simulink model "ADC_RoadRunner"  (R2024b)
settings: Solver=ode23tb  StartTime=0  StopTime=20  FixedStep=0.01  RelTol=1e-3
model workspace (MAT data in the model file):
  finalint = 0
  firstWarning = 1
  originalScenarioChecksum = '114339432DE22364D47BB28FC96DC10C'
undefined symbols (not defined in the file): curvature, DefaultGear, Defined, DEND_B, DEND_S, DEND_T, direction, DiscIntNeverNeededParam, driving, dspblkCoreblockFVToolHelper, Ego, fractalcoef, gcbh, gradbp, L, Lane, LF, LR, m, MAX_BRAKE, MAX_STEER, MAX_TORQUE, maxNumActors, MCAR, MIN_BRAKE, MIN_STEER, MIN_TORQUE, n, NUMD_B, NUMD_S, NUMD_T, Pose, psi_o, R, RRdamp, sigbuilder_block, STEER_RATIO, Tdead, thetaRefs, TrackWidth, ts, Ts, User, Vdead, Velocity, WB, xRef2s, yRef2s
libraries: simulink x9, roadrunnerscenario x7, simulink_extras x4, drivingscenarioandsensors x3, sensorinslib x2, robotalgslib x1, mpcadaslib x1, drivingvehiclecontroller x1, slpidlib x1, sensorgpslib x1, mspsensorlib x1, LaneDetection x1
(part 1 of 4)
settings Model: Creator=akshran  LastModifiedBy=austi
settings OptimizationCC: ReuseModelBlockBuffer=off
settings DebuggingCC: UnconnectedInputMsg=warning  UnconnectedOutputMsg=warning  UnconnectedLineMsg=warning  UnderSpecifiedDimensionMsg=warning
settings ModelReferenceCC: EnableRefExpFcnMdlSchedulingChecks=on
settings RTWCC: GPUComputeCapability=3.5  DLArmComputeVersion=19.05

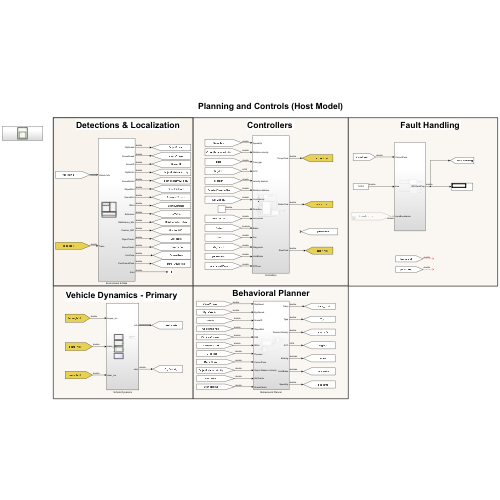
[thumbnail: Simulink's stored preview of the top-level diagram]
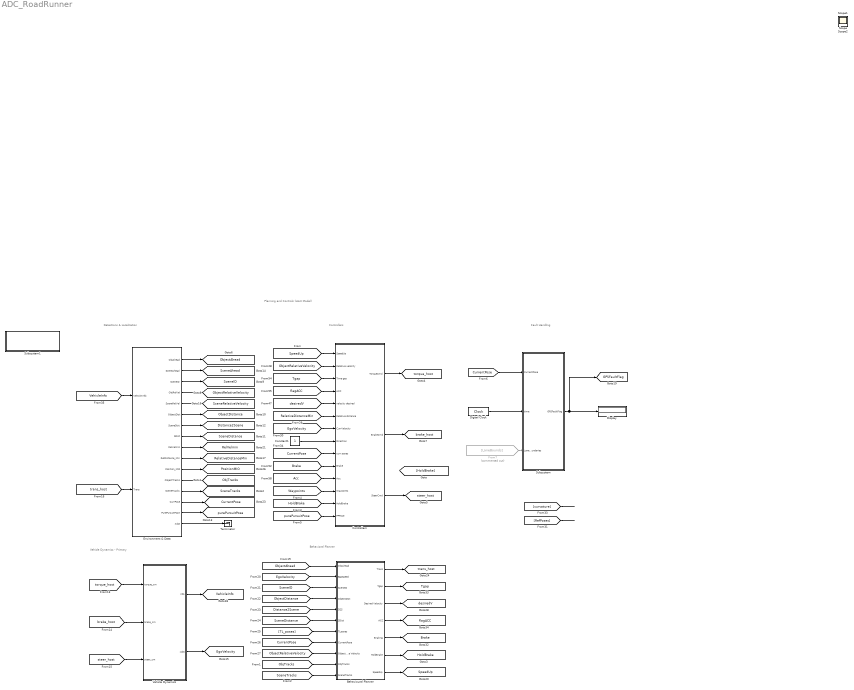
== system ADC_RoadRunner ==
  note: Planning and Controls (Host Model)
  note: Vehicle Dynamics - Primary
  note: Behavioral Planner
  note: Fault Handling
  note: Detections & Localization
  note: Controllers
  Behavioural Planner : Subsystem
  Constant1 : Constant
  Controllers : Subsystem
  Digital Clock : DigitalClock  SampleTime=Ts
  Display : Display
  Environment & Data : Subsystem
  From7 : From  Commented=on  GotoTag=LaneBounds  TagVisibility=global
  Subsystem : Subsystem
  Subsystem1 : Subsystem
  Terminator : Terminator
  Vehicle Dynamics : Subsystem
  Scope : Scope
  Scope1 : Scope
  Scope2 : Scope
  tag scope: Brake=global, CurrentPose=global, Distance2Scene=global, EgoVelocity=global, GPSFaultFlag=global, HoldBrake=global, ObjTracks=global, ObjectAhead=global, ObjectDistance=global, ObjectRelativeVelocity=global, PositionMIO=global, RelVelmin=global, RelativeDistanceMin=global, SceneAhead=global, SceneDistance=global, SceneID=global, SceneRelativeVelocity=global, SceneTracks=global, SpeedUp=global, Tgap=global, VehicleInfo=global, brake_host=global, desiredV=global, flagACC=global, purePursuitPose=global, steer_host=global, torque_host=global, trans_host=global
  wires:
  Controllers/1(TorqueCmd) -> [torque_host]
  Vehicle Dynamics/2(xdot) -> [EgoVelocity]
  Vehicle Dynamics/1(Info) -> [VehicleInfo]
  [torque_host] -> Vehicle Dynamics/1(torque_cm)
  [brake_host] -> Vehicle Dynamics/2(brake_cm)
  [steer_host] -> Vehicle Dynamics/3(steer_cm)
  [trans_host] -> Environment & Data/2(Trans)
  [ObjectRelativeVelocity] -> Controllers/2(Relative velocity)
  [RelativeDistanceMin] -> Controllers/6(Relative distance)
  [EgoVelocity] -> Controllers/7(CurrVelocity)
  [RefPoses] -> ?
  Constant1/1 -> Controllers/8(Direction)
  [curvature] -> ?
  [CurrentPose] -> Controllers/9(curr poses)
  [VehicleInfo] -> Environment & Data/1(Vehicle Info)
  [desiredV] -> Controllers/5(velocity desired)
  [Tgap] -> Controllers/3(Time gap)
  [flagACC] -> Controllers/4(ACC)
  Controllers/2(BrakeCmd) -> [brake_host]
  Controllers/3(SteerCmd) -> [steer_host]
  [ObjectAhead] -> Behavioural Planner/1(ObjAhead)
  [EgoVelocity] -> Behavioural Planner/2(EgoSpeed)
  [SceneID] -> Behavioural Planner/3(SceneID)
  [ObjectDistance] -> Behavioural Planner/4(ObjectDist)
  [Distance2Scene] -> Behavioural Planner/5(D2S)
  [SceneDistance] -> Behavioural Planner/6(SDist)
  [TL_poses] -> Behavioural Planner/7(TLposes)
  [CurrentPose] -> Behavioural Planner/8(CurrentPose)
  [ObjectRelativeVelocity] -> Behavioural Planner/9(Object Relative Velocity)
  Behavioural Planner/1(Trans) -> [trans_host]
  Behavioural Planner/2(Tgap) -> [Tgap]
  Behavioural Planner/3(Desired Velocity) -> [desiredV]
  Behavioural Planner/4(ACC) -> [flagACC]
  Behavioural Planner/5(Braking) -> [Brake]
  [Brake] -> Controllers/10(Brake)
  [Acc] -> Controllers/11(Acc)
  [ObjTracks] -> Behavioural Planner/10(ObjTracks)
  [SceneTracks] -> Behavioural Planner/11(SceneTracks)
  Behavioural Planner/6(HoldBrake) -> [HoldBrake]
  [HoldBrake] -> Controllers/13(HoldBrake)
  [Waypoints] -> Controllers/12(Waypoints)
  Behavioural Planner/7(SpeedUp) -> [SpeedUp]
  [SpeedUp] -> Controllers/1(SpeedUp)
  [purePursuitPose] -> Controllers/14(PPPose)
  [CurrentPose] -> Subsystem/1(CurrentPose)
  Digital Clock/1 -> Subsystem/2(time)
  Subsystem/1(GPSFaultFlag) -> Display/1, [GPSFaultFlag]
  Environment & Data/1(ObjAhead) -> [ObjectAhead]
  Environment & Data/4(ObjRelVel) -> [ObjectRelativeVelocity]
  Environment & Data/3(SceneID) -> [SceneID]
  Environment & Data/6(ObjectDist) -> [ObjectDistance]
  Environment & Data/7(SceneDist) -> [Distance2Scene]
  Environment & Data/8(SDist) -> [SceneDistance]
  Environment & Data/10(RelDistance_Min) -> [RelativeDistanceMin]
  Environment & Data/15(PurePursuitPose) -> [purePursuitPose]
  Environment & Data/14(CurrPose) -> [CurrentPose]
  Environment & Data/12(ObjectTracks) -> [ObjTracks]
  Environment & Data/13(SceneTracks) -> [SceneTracks]
  Environment & Data/11(Position_MIO) -> [PositionMIO]
  Environment & Data/2(SceneAhead) -> [SceneAhead]
  Environment & Data/9(RelVelmin) -> [RelVelmin]
  Environment & Data/5(SceneRelVel) -> [SceneRelativeVelocity]
  Environment & Data/16(Xdot) -> Terminator/1
  From7/1 -> Subsystem/3(LaneBoundaries)

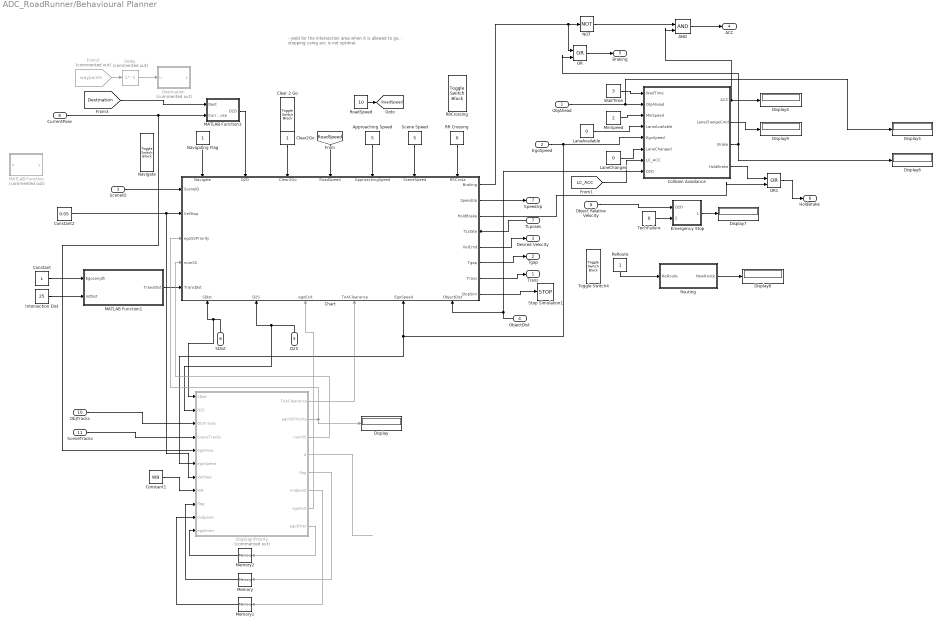
== system ADC_RoadRunner/Behavioural Planner ==
  note: - yield for the intersection area when it is allowed to go.
      | - stopping using acc is not optimal.
  ObjAhead : Inport
  EgoSpeed : Inport  Port=2
  SceneID : Inport  Port=3
  ObjectDist : Inport  Port=4
  D2S : Inport  Port=5
  SDist : Inport  Port=6
  TLposes : Inport  Port=7
  CurrentPose : Inport  Port=8
  Object Relative Velocity : Inport  Port=9
  ObjTracks : Inport  Port=10
  SceneTracks : Inport  Port=11
  AND : Logic  IconShape=distinctive  AllPortsSameDT=off  OutDataTypeStr=fixdt(1,16)
  Approaching Speed : Constant  Value=5
  Chart : Stateflow chart  TreatAsAtomicUnit=on
      settings: PortSchema="{\"entries\":[{\"content\":{\"sides\":[{\"content\":{\"connectorIds\":[\"In17\",\"In18\",\"In19\",\"In2\",\"In5\"]},\"type\":\"ConnectorPlacement.EquallySpacedRectSide\",\"uuid\":\"81aca70f-0947-49fb-b60a-be241e44193b\"},{\"content\":{\"connectorIds\":[\"Out6\",\"Out7\",\"Out2\",\"In1\",\"Out1\",\"Out3\",\"Out4\",\"Out5\"],\"side\":\"RIGHT\"},\"type\":\"ConnectorPlacement.EquallySpacedRectSide\",\"uuid\":\"e7b9645e-3711-4964-ac9b-0199dd335e99\"},{\"content\":{\"connectorIds\":[\"In13\",\"In14\",\"In15\",\"In16\",\"In6\",\"In9\",\"In11\"],\"side\":\"TOP\"},\"type\":\"ConnectorPlacement.EquallySpacedRectSide\",\"uuid\":\"6876f024-944b-4540-9404-d68f37763657\"},{\"content\":{\"connectorIds\":[\"In10\",\"In12\",\"In3\",\"In4\",\"In7\",\"In8\"],\"side\":\"BOTTOM\"},\"type\":\"ConnectorPlacement.EquallySpacedRectSide\",\"uuid\":\"44acab73-cdde-4edf-95df-27422644ccab\"}]},\"type\":\"ConnectorPlacement.EquallySpacedConnector\",\"uuid\":\"d2c31c01-e447-43db-8d2b-8b98a0ca291a\"}],\"packageUris\":[\"http://schema.mathworks.com/mf0/Connector/R2020b\"],\"version\":\"1.0\"}"
  Clear 2 Go : ToggleSwitchBlock
      settings: Values={{'Off', 'On'}, [0 1]}
  Clear2Go : Constant
  Collision Avoidance : Stateflow chart  TreatAsAtomicUnit=on
  Constant : Constant  Value=L
  Constant1 : Constant  Value=WB
  Constant2 : Constant  Value=0.05
  Delay : Delay  Commented=on  DelayLength=1
  Destination : MATLAB Function  Commented=on  TreatAsAtomicUnit=on
  Display{,4..9} (7 alike) : Display
  Emergency Stop : Stateflow chart  TreatAsAtomicUnit=on
  From2 : From  Commented=on  GotoTag=waypoints  TagVisibility=global
  Intersection Dist : Constant  Value=25
  LaneAvailable : Constant  Value=0
  LaneChanged : Constant  Value=0
  MATLAB Function : MATLAB Function  Commented=on  TreatAsAtomicUnit=on
  MATLAB Function1 : MATLAB Function  TreatAsAtomicUnit=on
  MATLAB Function3 : MATLAB Function  TreatAsAtomicUnit=on
  Memory : Memory
  Memory1 : Memory  InitialCondition=[0 0]
  Memory2 : Memory
  MinSpeed : Constant  Value=2
  NOT : Logic  Operator=NOT  IconShape=distinctive  AllPortsSameDT=off  OutDataTypeStr=boolean
  Navigate : ToggleSwitchBlock
      settings: Values={{'Off', 'On'}, [0 1]}
  Navigating Flag : Constant
  OR : Logic  Operator=OR  IconShape=distinctive  AllPortsSameDT=off  OutDataTypeStr=boolean
  OR1 : Logic  Operator=OR  IconShape=distinctive  AllPortsSameDT=off  OutDataTypeStr=boolean
  RR Crossing : Constant  Value=0
  RRCrossing : ToggleSwitchBlock
      settings: Values={{'Off', 'On'}, [0 1]}
  ReRoute : Constant
  RoadSpeed : Constant  Value=10
  Routing : Stateflow chart  TreatAsAtomicUnit=on
  Scene Speed : Constant  Value=5
  Stop Simulation1 : Stop
  StopSignPriority : MATLAB Function  Commented=on  TreatAsAtomicUnit=on
  TechFailure : Constant  Value=0
  Toggle Switch4 : ToggleSwitchBlock
      settings: Values={{'Off', 'On'}, [0 1]}
  WaitTime : Constant  Value=3
  Trans : Outport
  Tgap : Outport  Port=2
  Desired Velocity : Outport  Port=3
  ACC : Outport  Port=4
  Braking : Outport  Port=5
  HoldBrake : Outport  Port=6
  SpeedUp : Outport  Port=7
  tag scope: RoadSpeed=global
  wires:
  Clear2Go/1 -> Chart/15(Clear2Go)
  Routing/1(NewRoute) -> Display8/1
  ObjectDist/1 -> Chart/8(ObjectDist), Collision Avoidance/8(D2O)
  WaitTime/1 -> Collision Avoidance/1(WaitTime)
  Navigating Flag/1 -> Chart/13(Navigate)
  Approaching Speed/1 -> Chart/6(ApproachingSpeed)
  Scene Speed/1 -> Chart/9(SceneSpeed)
  EgoSpeed/1 -> Collision Avoidance/5(EgoSpeed), StopSignPriority/6(egoSpeed), Chart/7(EgoSpeed)
  ReRoute/1 -> Routing/1(ReRoute)
  Collision Avoidance/2(LaneChangeCmd) -> Display9/1
  LaneAvailable/1 -> Collision Avoidance/4(LaneAvailable)
  CurrentPose/1 -> StopSignPriority/5(egoPose), MATLAB Function3/2(CurrentPose)
  RR Crossing/1 -> Chart/11(RRCross)
  MinSpeed/1 -> Collision Avoidance/3(MinSpeed)
  LaneChanged/1 -> Collision Avoidance/6(LaneChanged)
  [RoadSpeed] -> Chart/16(RoadSpeed)
  ObjAhead/1 -> Display5/1, Collision Avoidance/2(ObjAhead)
  SceneID/1 -> Chart/17(SceneID)
  Chart/5(StopSim) -> Stop Simulation1/1
  Chart/4(Trans) -> Trans/1
  TLposes/1 -> Chart/1(TLstate)
  Chart/1(VelCmd) -> Desired Velocity/1
  SDist/1 -> Chart/10(SDist), StopSignPriority/1(SDist)
  D2S/1 -> Chart/12(D2S), StopSignPriority/2(D2S)
  Chart/3(Tgap) -> Tgap/1
  TechFailure/1 -> Emergency Stop/2(TechFailure)
  Emergency Stop/1(EStop) -> Display7/1
  Object Relative Velocity/1 -> Emergency Stop/1(D2O)
  Collision Avoidance/1(ACC) -> AND/2, Display4/1
  RoadSpeed/1 -> [RoadSpeed]
  NOT/1 -> AND/1
  AND/1 -> ACC/1
  Chart/6(Braking) -> OR/1, NOT/1
  OR/1 -> Braking/1
  Collision Avoidance/3(Brake) -> OR/2, Display6/1
  Constant/1 -> MATLAB Function1/1(EgoLength)
  Intersection Dist/1 -> MATLAB Function1/2(IntDist)
  MATLAB Function1/1(TransDist) -> Chart/5(TransDist)
  [LC_ACC] -> Collision Avoidance/7(LC_ACC)
  From2/1 -> Delay/1
  Delay/1 -> Destination/1(u)
  MATLAB Function3/1(D2D) -> Chart/14(D2D)
  Constant2/1 -> StopSignPriority/7(VelStop), Chart/18(VelStop)
  StopSignPriority/2(egoSSPriority) -> Display/1, Chart/19(egoSSPriority)
  SceneTracks/1 -> StopSignPriority/4(SceneTracks)
  ObjTracks/1 -> StopSignPriority/3(ObjTracks)
  StopSignPriority/3(numSS) -> Chart/2(numSS)
  Constant1/1 -> StopSignPriority/8(WB)
  StopSignPriority/4(d) -> ?
  Memory/1 -> StopSignPriority/9("flag ")
  StopSignPriority/5(flag) -> Memory/1
  StopSignPriority/6(midpoint) -> Memory1/1
  Memory1/1 -> StopSignPriority/10("midpoint ")
  StopSignPriority/7(egoExit) -> Chart/3(egoExit)
  StopSignPriority/1(ToAClearance) -> Chart/4(ToAClearance)
  Chart/2(HoldBrake) -> OR1/2
  StopSignPriority/8(egoEnter) -> Memory2/1
  Memory2/1 -> StopSignPriority/11("egoEnter ")
  OR1/1 -> HoldBrake/1
  Collision Avoidance/4(HoldBrake) -> OR1/1
  [Destination] -> MATLAB Function3/1(Dest)
  Chart/7(SpeedUp) -> SpeedUp/1

== system ADC_RoadRunner/Controllers ==
  SpeedUp : Inport
  Relative velocity : Inport  Port=2
  Time gap : Inport  Port=3
  ACC : Inport  Port=4
  velocity desired : Inport  Port=5
  Relative distance : Inport  Port=6
  CurrVelocity : Inport  Port=7
  Direction : Inport  Port=8
  curr poses : Inport  Port=9
  Brake : Inport  Port=10
  Acc : Inport  Port=11
  Waypoints : Inport  Port=12
  HoldBrake : Inport  Port=13
  PPPose : Inport  Port=14
  Lateral Controllers1 : Subsystem
  Longitudinal Controllers : Subsystem
  Steer Cmd : Display
  Subsystem2 : Subsystem
      settings: PortSchema="{\"entries\":[{\"content\":{\"sides\":[{\"content\":{\"connectorIds\":[\"In1\",\"In2\",\"In3\",\"In4\"]},\"type\":\"ConnectorPlacement.EquallySpacedRectSide\",\"uuid\":\"a23b1a10-3bcb-40a0-900c-c9a3f160b173\"},{\"content\":{\"connectorIds\":[\"Out1\",\"Out2\"],\"side\":\"RIGHT\"},\"type\":\"ConnectorPlacement.EquallySpacedRectSide\",\"uuid\":\"88840b66-912f-4184-aeec-297642319416\"},{\"content\":{\"connectorIds\":[\"In5\",\"In6\",\"In7\",\"In8\"],\"side\":\"TOP\"},\"type\":\"ConnectorPlacement.EquallySpacedRectSide\",\"uuid\":\"37a03ca9-b065-473e-b290-3b07703c6005\"},{\"content\":{\"connectorIds\":[\"In9\",\"In10\"],\"side\":\"BOTTOM\"},\"type\":\"ConnectorPlacement.EquallySpacedRectSide\",\"uuid\":\"275ca825-7815-497a-af18-67b3ec4705b4\"}]},\"type\":\"ConnectorPlacement.EquallySpacedConnector\",\"uuid\":\"5bfc7c71-8f7a-4cba-a168-7eeca22a2fcb\"}],\"packageUris\":[\"http://schema.mathworks.com/mf0/Connector/R2020b\"],\"version\":\"1.0\"}"
  Vector Concatenate : Concatenate  NumInputs=3
  TorqueCmd : Outport
  BrakeCmd : Outport  Port=2
  SteerCmd : Outport  Port=3
  wires:
  Acc/1 -> Subsystem2/9(CurrAccel), Longitudinal Controllers/11(Current Accel)
  velocity desired/1 -> Subsystem2/4(Set Velocity), Longitudinal Controllers/9(desiredVelocity), Longitudinal Controllers/5(Set velocity)
  Direction/1 -> Longitudinal Controllers/7(Direction)
  ACC/1 -> Subsystem2/5(ACC)
  PPPose/1 -> Lateral Controllers1/2(Pose)
  Brake/1 -> Subsystem2/8(Braking), Longitudinal Controllers/12(Brake)
  HoldBrake/1 -> Subsystem2/10(HoldBrake), Longitudinal Controllers/13(HoldBrake)
  curr poses/1 -> Longitudinal Controllers/10(CurrentPose)
  CurrVelocity/1 -> Subsystem2/6(CurrVelocity), Longitudinal Controllers/1(Curr Velocity), Longitudinal Controllers/6(CurrVel)
  Time gap/1 -> Longitudinal Controllers/4(Time gap)
  Relative distance/1 -> Subsystem2/7(Relative Distance), Longitudinal Controllers/3(Relative distance)
  Waypoints/1 -> Longitudinal Controllers/8(RefXY), Lateral Controllers1/1(Waypoints)
  Relative velocity/1 -> Longitudinal Controllers/2(Relative velocity)
  SpeedUp/1 -> Longitudinal Controllers/14(SpeedUp)
  Lateral Controllers1/1(steerCmd) -> SteerCmd/1, Steer Cmd/1
  Longitudinal Controllers/1(Longitudinal acceleration) -> Subsystem2/1(ACCaccel_cmd)
  Longitudinal Controllers/2(AccelCmd) -> Subsystem2/2(LCaccel_cmd)
  Longitudinal Controllers/3(DecelCmd) -> Subsystem2/3(LCdeccel_cmd)
  Subsystem2/1(TorqueCm) -> TorqueCmd/1
  Subsystem2/2(BrakeCm) -> Vector Concatenate/2, BrakeCmd/1

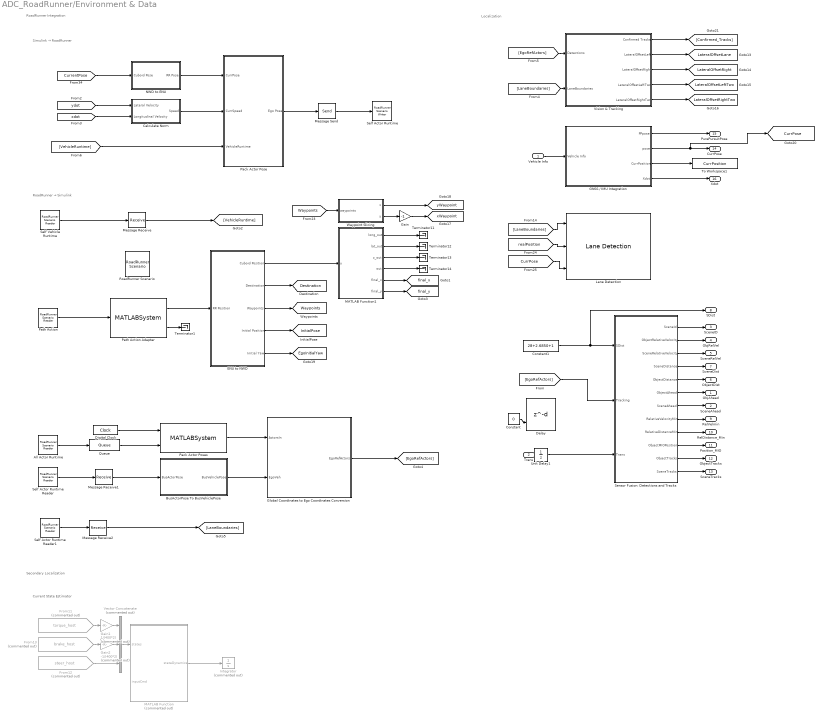
== system ADC_RoadRunner/Environment & Data ==
  note: RoadRunner Integration
  note: Simulink → RoadRunner
  note: RoadRunner → Simulink
  note: Localization
  note: Secondary Localization
  note: Current State Estimator
  Vehicle Info : Inport
  Trans : Inport  Port=2
  All Actor Runtime : roadrunnerscenario/RoadRunner Scenario Reader  TopicCategory=Actor  ActorCategory=All Types  ActionType=Path Following  EventType=User-Defined  TopicType=Actor Pose (Driving Scenario compatible)  VehicleType=Vehicle Specifications  UserDefinedAction=Action1  UserDefinedEvent=Event1  Filter=None  SensorTopic=Target Poses  LaneBoundaryOutputTopic=Ego-Lane  SensorID=1  SampleTime=Ts
  BusActorPose To BusVehiclePose : Subsystem
  Calculate Norm : Subsystem
  Constant : Constant  Value=0
  Constant1 : Constant  Value=28+2.6850+1
  Delay : Delay  DelayLengthSource=Input port
      settings: InputPortMap=u0,p1
  Digital Clock : DigitalClock  SampleTime=Ts
  ENU to NWD : Subsystem
  From11 : From  Commented=on  GotoTag=torque_host  TagVisibility=global
  From12 : From  Commented=on  GotoTag=steer_host  TagVisibility=global
  From13 : From  Commented=on  GotoTag=brake_host  TagVisibility=global
  GNSS / IMU Integration : Subsystem
  Gain : Gain  Gain=-1
  Gain1 : Gain  Commented=on  Gain=1/(400*2)
  Gain2 : Gain  Commented=on  Gain=-1/(400*2)
  Global Coordinates to Ego Coordinates Conversion : MATLAB Function  TreatAsAtomicUnit=on
  Integrator : Integrator  Commented=on
  Lane Detection : LaneDetection/Lane Detection  SystemSampleTime=-1  VariantActivationTime=update diagram  AllowFlexibleInterface=on  Latency=0  AutoFrameSizeCalculation=off
  MATLAB Function : MATLAB Function  Commented=on  TreatAsAtomicUnit=on
  MATLAB Function1 : MATLAB Function  TreatAsAtomicUnit=on
  Message Receive : Receive  InputPortMessageModes=m
  Message Receive1 : Receive  InputPortMessageModes=m  SampleTime=Ts
  Message Receive2 : Receive  InputPortMessageModes=m  UseInternalQueue=off  SampleTime=Ts
  Message Send : Send  OutputPortMessageModes=m
  NWD to ENU : Subsystem
  Pack Actor Pose : Subsystem
  Pack Actor Poses : MATLABSystem  InputPortMessageModes=n,m  System=HelperPackDrivingScenarioPoses  EgoActorID=1  ActorProfiles=struct( 'ActorID', 1, 'ClassID', 1, 'Length', 4.7, 'Width', 1.8, 'Height', 1.4, 'OriginOffset', [ 0, 0, 0 ], 'FrontOverhang', 0, 'RearOverhang', 0, 'Wheelbase', 0, 'Color', [ 0, 0, 0 ] )  DefaultActorPoses="Simulink.Bus.createMATLABStruct( \"BusActors\" )"
      mask Type: HelperPackDrivingScenarioPoses
      mask Display:
      | disp(['HelperPack' char(10) 'DrivingScenarioPoses']);
      | port_label('input',1,'time');
      | port_label('input',2,'msgs');
      | port_label('output',1,'TargetPoses');
  Path Action : roadrunnerscenario/RoadRunner Scenario Reader  TopicCategory=Action  ActorCategory=All Types  ActionType=Path Following  EventType=User-Defined  TopicType=Actor Specifications  VehicleType=Vehicle Specifications  UserDefinedAction=Action1  UserDefinedEvent=Event1  Filter=Self  SensorTopic=Target Poses  LaneBoundaryOutputTopic=Ego-Lane  SensorID=1  SampleTime=Ts
  Path Action Adapter : MATLABSystem  InputPortMessageModes=m  System=HelperPathActionAdapter
      mask Type: HelperPathActionAdapter
      mask Display:
      | disp(['HelperPathActionAdapter' char(10) '' char(10) '']);
      | port_label('input',1,'PathAction');
      | port_label('output',1,'Path');
      | port_label('output',2,'NumPoints');
  Queue : Queue  InputPortMessageModes=m  OutputPortMessageModes=m  OverwriteOldest=on  Capacity=maxNumActors+1
  RoadRunner Scenario : roadrunnerscenario/RoadRunner Scenario  UserDefinedActions={}  UserDefinedEvents={}
  Self Actor Runtime : roadrunnerscenario/RoadRunner Scenario Writer  TopicCategory=Actor  ActorCategory=All Types  EventType=Action Complete  UserDefinedEvent=Event1  VehicleType=Vehicle Pose  TopicType=Actor Pose
  Self Actor Runtime Reader : roadrunnerscenario/RoadRunner Scenario Reader  TopicCategory=Actor  ActorCategory=All Types  ActionType=Path Following  EventType=User-Defined  TopicType=Actor Pose (Driving Scenario compatible)  VehicleType=Vehicle Specifications  UserDefinedAction=Action1  UserDefinedEvent=Event1  Filter=Self  SensorTopic=Target Poses  LaneBoundaryOutputTopic=Ego-Lane  SensorID=1  SampleTime=Ts
  Self Actor Runtime Reader1 : roadrunnerscenario/RoadRunner Scenario Reader  TopicCategory=Sensor  ActorCategory=All Types  ActionType=Lateral Offset  EventType=User-Defined  TopicType=Actor Lane Location  VehicleType=Vehicle Specifications  UserDefinedAction=Action1  UserDefinedEvent=Event1  Filter=Self  SensorTopic=Lane Boundaries  LaneBoundaryOutputTopic=Ego and Adjacent Lanes  SensorID=1  SampleTime=Ts
  Self Vehicle Runtime : roadrunnerscenario/RoadRunner Scenario Reader  TopicCategory=Actor  ActorCategory=Vehicle  ActionType=Path Following  EventType=User-Defined  TopicType=Actor Specifications  VehicleType=Vehicle Pose  UserDefinedAction=Action1  UserDefinedEvent=Event1  Filter=Self  SensorTopic=Target Poses  LaneBoundaryOutputTopic=Ego-Lane  SensorID=1  SampleTime=Ts
  Sensor Fusion: Detections and Tracks : MATLAB Function  TreatAsAtomicUnit=on
  Terminator{1,11..14} (5 alike) : Terminator
  To Workspace1 : ToWorkspace  VariableName=CurrPosition  SaveFormat=Structure  SampleTime=-1
      settings: Save2DSignal=2-D array (concatenate along first dimension)
  Unit Delay1 : UnitDelay  SampleTime=0.05  HasFrameUpgradeWarning=on
  Vector Concatenate : Concatenate  Commented=on  NumInputs=3
  Vision & Tracking : Subsystem
  Waypoint Slicing : MATLAB Function  TreatAsAtomicUnit=on
  ObjAhead : Outport
  SceneAhead : Outport  Port=2
  SceneID : Outport  Port=3
  ObjRelVel : Outport  Port=4
  SceneRelVel : Outport  Port=5
  ObjectDist : Outport  Port=6
  SceneDist : Outport  Port=7
  SDist : Outport  Port=8
  RelVelmin : Outport  Port=9
  RelDistance_Min : Outport  Port=10
  Position_MIO : Outport  Port=11
  ObjectTracks : Outport  Port=12
  SceneTracks : Outport  Port=13
  CurrPose : Outport  Port=14
  PurePursuitPose : Outport  Port=15
  Xdot : Outport  Port=16
  tag scope: CurrPose=global, Destination=global, EgoInitialYaw=global, InitialPose=global, LateralOffsetLane=global, LateralOffsetLeftTwo=global, LateralOffsetRight=global, LateralOffsetRightTwo=global, Waypoints=global, final_x=global, final_y=global, xWaypoint=global, yWaypoint=global
  wires:
  Vehicle Info/1 -> GNSS / IMU Integration/1(Vehicle Info)
  [CurrentPose] -> NWD to ENU/1(Cuboid Pose)
  MATLAB Function1/6(final_y) -> [final_y]
  Sensor Fusion: Detections and Tracks/9(RelativeDistanceMin) -> RelDistance_Min/1
  Path Action Adapter/1 -> ENU to NWD/1(RR Position)
  ENU to NWD/3(Waypoints) -> [Waypoints]
  Path Action/1 -> Path Action Adapter/1
  Trans/1 -> Unit Delay1/1
  Calculate Norm/1(Speed) -> Pack Actor Pose/2(CurrSpeed)
  Sensor Fusion: Detections and Tracks/3(SceneRelativeVelocity) -> SceneRelVel/1
  GNSS / IMU Integration/2(pose) -> [CurrPose], CurrPose/1
  Sensor Fusion: Detections and Tracks/2(ObjectRelativeVelocity) -> ObjRelVel/1
  MATLAB Function1/1(long_out) -> Terminator11/1
  Sensor Fusion: Detections and Tracks/10(ObjectMIOPosition) -> Position_MIO/1
  GNSS / IMU Integration/3(CurrPosition) -> To Workspace1/1
  ENU to NWD/1(Cuboid Position) -> MATLAB Function1/1(u)
  MATLAB Function1/2(lat_out) -> Terminator12/1
  ENU to NWD/2(Destination) -> [Destination]
  Constant/1 -> Delay/2
  Constant1/1 -> SDist/1, Sensor Fusion: Detections and Tracks/1(SDist)
  Message Receive/1 -> [VehicleRuntime]
  ENU to NWD/4(Initial Position) -> [InitialPose]
  NWD to ENU/1(RR Pose) -> Pack Actor Pose/1(CurrPose)
  Sensor Fusion: Detections and Tracks/12(SceneTracks) -> SceneTracks/1
  Sensor Fusion: Detections and Tracks/8(RelativeVelocityMin) -> RelVelmin/1
  Self Vehicle Runtime/1 -> Message Receive/1
  Sensor Fusion: Detections and Tracks/5(ObjectDistance) -> ObjectDist/1
  MATLAB Function1/3(z_out) -> Terminator13/1
  [xdot] -> Calculate Norm/2(Longitudinal Velocity)
  MATLAB Function1/5(final_x) -> [final_x]
  Unit Delay1/1 -> Sensor Fusion: Detections and Tracks/3(Trans)
  [VehicleRuntime] -> Pack Actor Pose/3(VehicleRuntime)
  MATLAB Function1/4(out) -> Terminator14/1
  Sensor Fusion: Detections and Tracks/7(SceneAhead) -> SceneAhead/1
  Sensor Fusion: Detections and Tracks/6(ObjectAhead) -> ObjAhead/1
  Message Send/1 -> Self Actor Runtime/1
  [ydot] -> Calculate Norm/1(Lateral Velocity)
  GNSS / IMU Integration/4(Xdot) -> Xdot/1
  Sensor Fusion: Detections and Tracks/4(SceneDistance) -> SceneDist/1
  Sensor Fusion: Detections and Tracks/11(ObjectTracks) -> ObjectTracks/1
  Sensor Fusion: Detections and Tracks/1(SceneId) -> SceneID/1
  [EgoRefActors] -> Sensor Fusion: Detections and Tracks/2(Tracking)
  Pack Actor Pose/1(Ego Pose) -> Message Send/1
  Vision & Tracking/1(Confirmed Tracks) -> [Confirmed_Tracks]
  Message Receive1/1 -> BusActorPose To BusVehiclePose/1(BusActorPose)
  Self Actor Runtime Reader/1 -> Message Receive1/1
  Digital Clock/1 -> Pack Actor Poses/1
  Queue/1 -> Pack Actor Poses/2
  BusActorPose To BusVehiclePose/1(BusVehiclePose) -> Global Coordinates to Ego Coordinates Conversion/2(EgoVeh)
  All Actor Runtime/1 -> Queue/1
  Pack Actor Poses/1 -> Global Coordinates to Ego Coordinates Conversion/1(ActorsIn)
  Global Coordinates to Ego Coordinates Conversion/1(EgoRefActors) -> [EgoRefActors]
  [EgoRefActors] -> Vision & Tracking/1(Detections)
  Self Actor Runtime Reader1/1 -> Message Receive2/1
  Message Receive2/1 -> [LaneBoundaries]
  [LaneBoundaries] -> Vision & Tracking/2(LaneBoundaries)
  Path Action Adapter/2 -> Terminator1/1
  [LaneBoundaries] -> Lane Detection/1
  MATLAB Function/1(stateDynamics) -> Integrator/1
  From11/1 -> Gain1/1
  From12/1 -> Vector Concatenate/3
  Vector Concatenate/1 -> MATLAB Function/1(states)
  From13/1 -> Gain2/1
  Gain1/1 -> Vector Concatenate/1
  Gain2/1 -> Vector Concatenate/2
  ? -> ?
  Vision & Tracking/2(LateralOffsetLeft) -> [LateralOffsetLane]
  Vision & Tracking/3(LateralOffsetRight) -> [LateralOffsetRight]
  Vision & Tracking/4(LateralOffsetLeftTwo) -> [LateralOffsetLeftTwo]
  Vision & Tracking/5(LateralOffsetRightTwo) -> [LateralOffsetRightTwo]
  Gain/1 -> [xWaypoint]
  ENU to NWD/5(Initial Yaw) -> [EgoInitialYaw]
  [Waypoints] -> Waypoint Slicing/1(waypoints)
  Waypoint Slicing/1(x) -> [yWaypoint]
  Waypoint Slicing/2(y) -> Gain/1
  [realPosition] -> Lane Detection/2
  [CurrPose] -> Lane Detection/3
  GNSS / IMU Integration/1(PPpose) -> PurePursuitPose/1

== system ADC_RoadRunner/Subsystem ==
  CurrentPose : Inport
  time : Inport  Port=2
  LaneBoundaries : Inport  Port=3
  MATLAB Function : MATLAB Function  TreatAsAtomicUnit=on
  MATLAB Function4 : MATLAB Function  Commented=on  TreatAsAtomicUnit=on
  Terminator1 : Terminator
  Terminator2 : Terminator
  GPSFaultFlag : Outport
  wires:
  CurrentPose/1 -> MATLAB Function/1(CurrentPose)
  time/1 -> MATLAB Function/2(time)
  MATLAB Function/1(GPSFaultFlag) -> GPSFaultFlag/1
  MATLAB Function4/2(yrightLane) -> Terminator2/1
  MATLAB Function4/1(yleftLane) -> Terminator1/1
  LaneBoundaries/1 -> MATLAB Function4/1(Lanebounds)

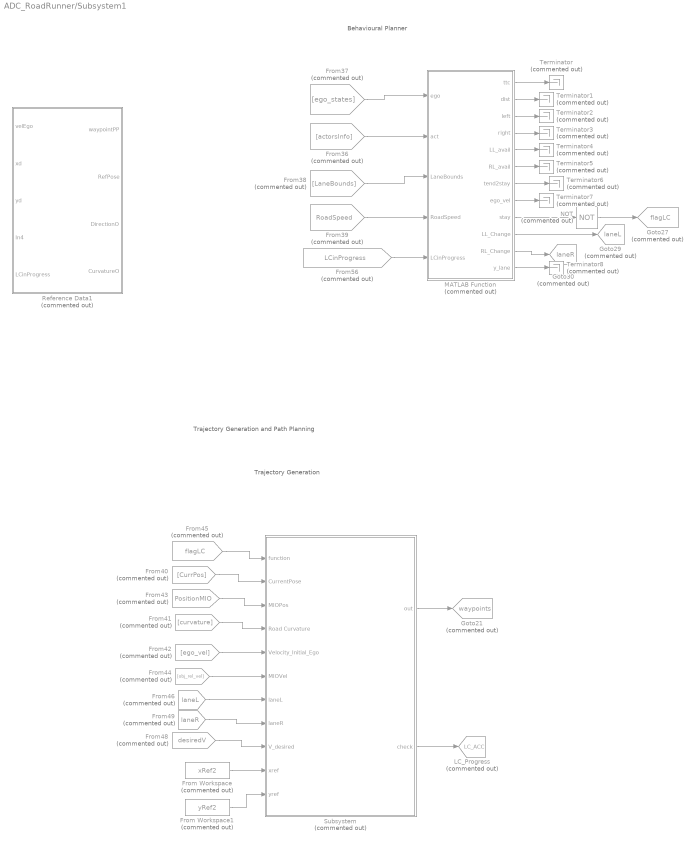
== system ADC_RoadRunner/Subsystem1 ==
  note: Trajectory Generation and Path Planning
  note: Trajectory Generation
  note: Behavioural Planner
  From Workspace : FromWorkspace  Commented=on  VariableName=xRef2
  From Workspace1 : FromWorkspace  Commented=on  VariableName=yRef2
  From36 : From  Commented=on  GotoTag=actorsInfo  TagVisibility=global
  From37 : From  Commented=on  GotoTag=ego_states  TagVisibility=global
  From38 : From  Commented=on  GotoTag=LaneBounds  TagVisibility=global
  From39 : From  Commented=on  GotoTag=RoadSpeed  TagVisibility=global
  From40 : From  Commented=on  GotoTag=CurrPos  TagVisibility=global
  From41 : From  Commented=on  GotoTag=curvature
  From42 : From  Commented=on  GotoTag=ego_vel  TagVisibility=global
  From43 : From  Commented=on  GotoTag=PositionMIO  TagVisibility=global
  From44 : From  Commented=on  GotoTag=obj_rel_vel  TagVisibility=global
  From45 : From  Commented=on  GotoTag=flagLC  TagVisibility=global
  From46 : From  Commented=on  GotoTag=laneL  TagVisibility=global
  From48 : From  Commented=on  GotoTag=desiredV  TagVisibility=global
  From49 : From  Commented=on  GotoTag=laneR  TagVisibility=global
  From56 : From  Commented=on  GotoTag=LCinProgress  TagVisibility=global
  Goto21 : Goto  Commented=on  GotoTag=waypoints  TagVisibility=global
  Goto27 : Goto  Commented=on  GotoTag=flagLC  TagVisibility=global
  Goto29 : Goto  Commented=on  GotoTag=laneL  TagVisibility=global
  Goto30 : Goto  Commented=on  GotoTag=laneR  TagVisibility=global
  LC_Progress : Goto  Commented=on  GotoTag=LC_ACC  TagVisibility=global
  MATLAB Function : MATLAB Function  Commented=on  TreatAsAtomicUnit=on
  NOT : Logic  Commented=on  Operator=NOT  IconShape=distinctive  AllPortsSameDT=off  OutDataTypeStr=boolean
  Reference Data1 : Subsystem  Commented=on  VariantControl=Stanley
  Subsystem : Subsystem  Commented=on
  Terminator{,1..8} (9 alike) : Terminator  Commented=on
  wires:
  MATLAB Function/12(y_lane) -> Terminator8/1
  From Workspace1/1 -> Subsystem/11(yref)
  MATLAB Function/10(LL_Change) -> Goto29/1
  From36/1 -> MATLAB Function/2(act)
  From39/1 -> MATLAB Function/4(RoadSpeed)
  From41/1 -> Subsystem/4(Road Curvature)
  Subsystem/1(out) -> Goto21/1
  MATLAB Function/2(dist) -> Terminator1/1
  From48/1 -> Subsystem/9(V_desired)
  MATLAB Function/1(ttc) -> Terminator/1
  From44/1 -> Subsystem/6(MIOVel)
  From42/1 -> Subsystem/5(Velocity_Initial_Ego)
  Subsystem/2(check) -> LC_Progress/1
  From49/1 -> Subsystem/8(laneR)
  From37/1 -> MATLAB Function/1(ego)
  MATLAB Function/6(RL_avail) -> Terminator5/1
  MATLAB Function/9(stay) -> NOT/1
  NOT/1 -> Goto27/1
  From40/1 -> Subsystem/2(CurrentPose)
  From56/1 -> MATLAB Function/5(LCinProgress)
  From Workspace/1 -> Subsystem/10(xref)
  MATLAB Function/4(right) -> Terminator3/1
  From45/1 -> Subsystem/1(function)
  MATLAB Function/5(LL_avail) -> Terminator4/1
  From46/1 -> Subsystem/7(laneL)
  From43/1 -> Subsystem/3(MIOPos)
  MATLAB Function/11(RL_Change) -> Goto30/1
  From38/1 -> MATLAB Function/3(LaneBounds)
  MATLAB Function/8(ego_vel) -> Terminator7/1
  MATLAB Function/7(tend2stay) -> Terminator6/1
  MATLAB Function/3(left) -> Terminator2/1

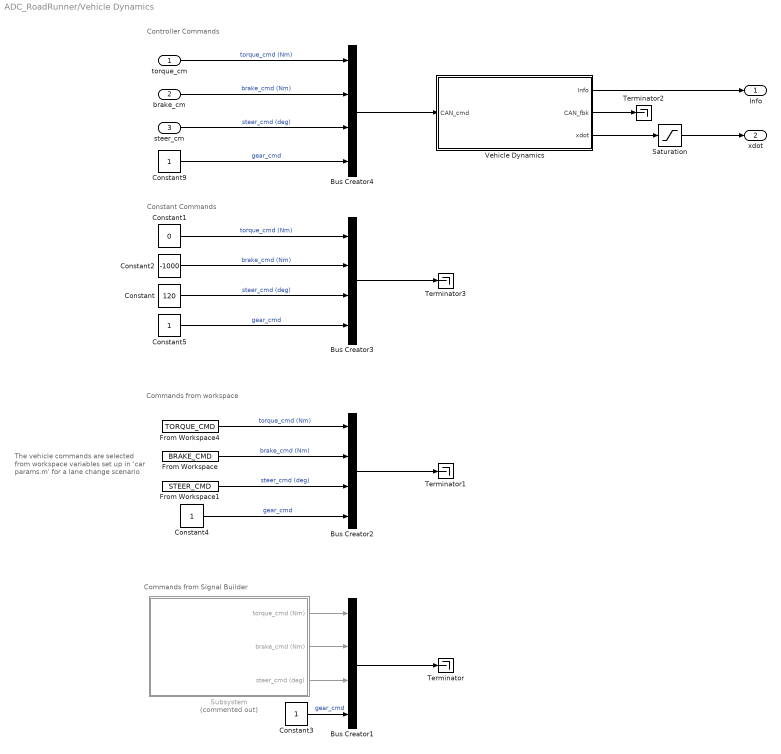
== system ADC_RoadRunner/Vehicle Dynamics ==
  note: Constant Commands
  note: Commands from workspace
  note: Commands from Signal Builder
  note: The vehicle commands are selected from workspace variables set up in 'car params.m' for a lane change scenario
  note: Controller Commands
  torque_cm : Inport
  brake_cm : Inport  Port=2
  steer_cm : Inport  Port=3
  Bus Creator{1..4} (4 alike) : BusCreator  Inputs=4
  Constant : Constant  Value=120
  Constant1 : Constant  Value=0
  Constant2 : Constant  Value=-1000
  Constant{3..5,9} (4 alike) : Constant
  From Workspace : FromWorkspace  VariableName=BRAKE_CMD  SampleTime=ts
  From Workspace1 : FromWorkspace  VariableName=STEER_CMD  SampleTime=ts
  From Workspace4 : FromWorkspace  VariableName=TORQUE_CMD  SampleTime=ts
  Saturation : Saturate  UpperLimit=inf  LowerLimit=0.001
  Subsystem : Subsystem  Commented=on
  Terminator{,1..3} (4 alike) : Terminator
  Vehicle Dynamics : Subsystem  mask{InitPosition=[0 0 0]*0, InitSpeed=0, InitYaw=0}
      mask prompts: InitPosition "Initial Position (m)"; InitSpeed "Initial Speed (m/s)"; InitYaw "Init Yaw (rad)"
  Info : Outport
  xdot : Outport  Port=2
  wires:
  Bus Creator2/1 -> Terminator1/1
  Vehicle Dynamics/2(CAN_fbk) -> Terminator2/1
  Vehicle Dynamics/1(Info) -> Info/1
  Constant/1 -> Bus Creator3/3  "steer_cmd (deg)"
  Constant1/1 -> Bus Creator3/1  "torque_cmd (Nm)"
  Constant2/1 -> Bus Creator3/2  "brake_cmd (Nm)"
  Vehicle Dynamics/3(xdot) -> Saturation/1
  Subsystem/1(torque_cmd (Nm)) -> Bus Creator1/1
  Subsystem/2(brake_cmd (Nm)) -> Bus Creator1/2
  Subsystem/3(steer_cmd (deg)) -> Bus Creator1/3
  Constant3/1 -> Bus Creator1/4  "gear_cmd"
  Constant4/1 -> Bus Creator2/4  "gear_cmd"
  From Workspace/1 -> Bus Creator2/2  "brake_cmd (Nm)"
  From Workspace1/1 -> Bus Creator2/3  "steer_cmd (deg)"
  From Workspace4/1 -> Bus Creator2/1  "torque_cmd (Nm)"
  Constant5/1 -> Bus Creator3/4  "gear_cmd"
  Bus Creator1/1 -> Terminator/1
  brake_cm/1 -> Bus Creator4/2  "brake_cmd (Nm)"
  Constant9/1 -> Bus Creator4/4  "gear_cmd"
  torque_cm/1 -> Bus Creator4/1  "torque_cmd (Nm)"
  steer_cm/1 -> Bus Creator4/3  "steer_cmd (deg)"
  Bus Creator3/1 -> Terminator3/1
  Bus Creator4/1 -> Vehicle Dynamics/1(CAN_cmd)
  Saturation/1 -> xdot/1

== system ADC_RoadRunner/Controllers/Lateral Controllers1 ==
  Waypoints : Inport
  Pose : Inport  Port=2
  Gain : Gain  Gain=1/STEER_RATIO
  Gain2 : Gain  Gain=180/pi
  Pure Pursuit Controller1 : Subsystem
  steerCmd : Outport
  wires:
  Pure Pursuit Controller1/1(delta) -> Gain2/1
  Gain/1 -> steerCmd/1
  Pose/1 -> Pure Pursuit Controller1/1(Pose)
  Gain2/1 -> Gain/1
  Waypoints/1 -> Pure Pursuit Controller1/2(Waypoints)

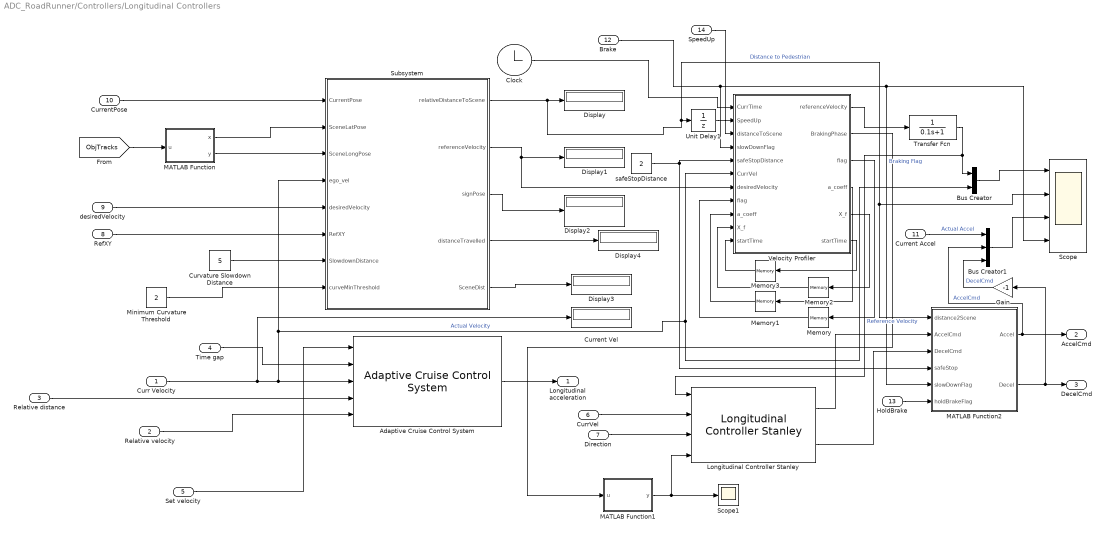
== system ADC_RoadRunner/Controllers/Longitudinal Controllers ==
  Curr Velocity : Inport
  Relative velocity : Inport  Port=2
  Relative distance : Inport  Port=3
  Time gap : Inport  Port=4
  Set velocity : Inport  Port=5
  CurrVel : Inport  Port=6
  Direction : Inport  Port=7
  RefXY : Inport  Port=8
  desiredVelocity : Inport  Port=9
  CurrentPose : Inport  Port=10
  Current Accel : Inport  Port=11
  Brake : Inport  Port=12
  HoldBrake : Inport  Port=13
  SpeedUp : Inport  Port=14
  Adaptive Cruise Control System : mpcadaslib/Adaptive Cruise Control System  EgoModel=tf(1,[0.5,1,0])  InitialEgoVelocity=0  DefaultSpacing=WB+2  MaxVelocity=50  MinAcceleration=-40  amin_ext=off  MaxAcceleration=40  amax_ext=off  Ts=0.1  PredictionHorizon=10  ControllerBehavior=1.0  suboptimal=off  maxiter=10  datatypeopt=double  optmode=off  trackmode=off
  Bus Creator : BusCreator  Inputs=2
  Bus Creator1 : BusCreator  Inputs=3
  Clock : Clock
  Current Vel : Display
  Curvature Slowdown Distance : Constant  Value=5
  Display{,1..4} (5 alike) : Display
  Gain : Gain  Gain=-1
  Longitudinal Controller Stanley : drivingvehiclecontroller/Longitudinal Controller Stanley  Kp=1.9  Ki=1.4  SampleTime=0.05  MaxAcceleration=3  MaxDeceleration=3
  MATLAB Function : MATLAB Function  TreatAsAtomicUnit=on
  MATLAB Function1 : MATLAB Function  TreatAsAtomicUnit=on
  MATLAB Function2 : MATLAB Function  TreatAsAtomicUnit=on
  Memory : Memory  InheritSampleTime=on
  Memory1 : Memory  InitialCondition=zeros(6,1)  InheritSampleTime=on
  Memory2 : Memory  InheritSampleTime=on
  Memory3 : Memory  InheritSampleTime=on
  "Minimum Curvature Threshold " : Constant  Value=2
  Scope : Scope  NumInputPorts=4
  Scope1 : Scope
  Subsystem : Subsystem
  Transfer Fcn : TransferFcn  Denominator=[0.1 1]
  Unit Delay1 : UnitDelay  SampleTime=-1  HasFrameUpgradeWarning=on
  Velocity Profiler : MATLAB Function  TreatAsAtomicUnit=on
  safeStopDistance : Constant  Value=2
  Longitudinal acceleration : Outport
  AccelCmd : Outport  Port=2
  DecelCmd : Outport  Port=3
  wires:
  Set velocity/1 -> Adaptive Cruise Control System/1
  Curr Velocity/1 -> Current Vel/1, Subsystem/4(ego_vel), Bus Creator/2, Velocity Profiler/6(CurrVel), Adaptive Cruise Control System/3  "Actual Velocity"
  CurrVel/1 -> Longitudinal Controller Stanley/2
  Longitudinal Controller Stanley/2 -> MATLAB Function2/3(DecelCmd)
  Relative velocity/1 -> Adaptive Cruise Control System/5
  Relative distance/1 -> Adaptive Cruise Control System/4
  Adaptive Cruise Control System/1 -> Longitudinal acceleration/1
  Time gap/1 -> Adaptive Cruise Control System/2
  Direction/1 -> Longitudinal Controller Stanley/3
  Curvature Slowdown Distance/1 -> Subsystem/7(SlowdownDistance)
  "Minimum Curvature Threshold "/1 -> Subsystem/8(curveMinThreshold)
  RefXY/1 -> Subsystem/6(RefXY)
  desiredVelocity/1 -> Subsystem/5(desiredVelocity)
  CurrentPose/1 -> Subsystem/1(CurrentPose)
  [ObjTracks] -> MATLAB Function/1(u)
  MATLAB Function/1(x) -> Subsystem/2(SceneLatPose)
  MATLAB Function/2(y) -> Subsystem/3(SceneLongPose)
  Subsystem/1(relativeDistanceToScene) -> Unit Delay1/1, MATLAB Function2/1(distance2Scene), Scope/2, Display/1  "Distance to Pedestrian"
  Subsystem/3(signPose) -> Display2/1
  Brake/1 -> Scope/4, MATLAB Function2/5(slowDownFlag), Velocity Profiler/4(slowDownFlag)  "Braking Flag"
  safeStopDistance/1 -> Velocity Profiler/5(safeStopDistance), MATLAB Function2/4(safeStop)
  Velocity Profiler/1(referenceVelocity) -> Transfer Fcn/1
  MATLAB Function2/2(Decel) -> Gain/1, DecelCmd/1
  MATLAB Function2/1(Accel) -> Bus Creator1/2, AccelCmd/1  "AccelCmd"
  Longitudinal Controller Stanley/1 -> MATLAB Function2/2(AccelCmd)
  Bus Creator/1 -> Scope/1
  Current Accel/1 -> Bus Creator1/1  "Actual Accel"
  Bus Creator1/1 -> Scope/3
  Gain/1 -> Bus Creator1/3  "DecelCmd"
  Transfer Fcn/1 -> Bus Creator/1, Longitudinal Controller Stanley/1  "Reference Velocity"
  Subsystem/2(referenceVelocity) -> Velocity Profiler/7(desiredVelocity), Display1/1
  Velocity Profiler/4(a_coeff) -> Memory1/1
  Memory1/1 -> Velocity Profiler/9("a_coeff ")
  Velocity Profiler/3(flag) -> Memory/1
  Memory/1 -> Velocity Profiler/8("flag ")
  Unit Delay1/1 -> Velocity Profiler/3(distanceToScene)
  Subsystem/5(SceneDist) -> Display3/1
  Velocity Profiler/2(BrakingPhase) -> MATLAB Function1/1(u)
  MATLAB Function1/1(y) -> Scope1/1, Longitudinal Controller Stanley/4
  HoldBrake/1 -> MATLAB Function2/6(holdBrakeFlag)
  SpeedUp/1 -> Velocity Profiler/2(SpeedUp)
  Subsystem/4(distanceTravelled) -> Display4/1
  Velocity Profiler/5(X_f) -> Memory2/1
  Memory2/1 -> Velocity Profiler/10("X_f ")
  Velocity Profiler/6(startTime) -> Memory3/1
  Memory3/1 -> Velocity Profiler/11("startTime ")
  Clock/1 -> Velocity Profiler/1(CurrTime)

== system ADC_RoadRunner/Controllers/Subsystem2 ==
  ACCaccel_cmd : Inport
  LCaccel_cmd : Inport  Port=2
  LCdeccel_cmd : Inport  Port=3
  Set Velocity : Inport  Port=4
  ACC : Inport  Port=5
  CurrVelocity : Inport  Port=6
  Relative Distance : Inport  Port=7
  Braking : Inport  Port=8
  CurrAccel : Inport  Port=9
  HoldBrake : Inport  Port=10
  Acceleration to Torque : Subsystem
  Braking Command : Subsystem
      settings: PortSchema="{\"entries\":[{\"content\":{\"sides\":[{\"content\":{\"connectorIds\":[\"In1\",\"In2\",\"In3\",\"In4\",\"In5\"]},\"type\":\"ConnectorPlacement.EquallySpacedRectSide\",\"uuid\":\"6c9a9437-5364-4180-a50b-e6d6b79cdde7\"},{\"content\":{\"connectorIds\":[\"Out1\"],\"side\":\"RIGHT\"},\"type\":\"ConnectorPlacement.EquallySpacedRectSide\",\"uuid\":\"0c9d90ab-7b55-4efa-a55f-4d6656a67f49\"},{\"content\":{\"side\":\"TOP\"},\"type\":\"ConnectorPlacement.EquallySpacedRectSide\",\"uuid\":\"ae5230ee-a902-425c-beff-008108cd3a63\"},{\"content\":{\"connectorIds\":[\"In6\"],\"side\":\"BOTTOM\"},\"type\":\"ConnectorPlacement.EquallySpacedRectSide\",\"uuid\":\"84107842-f68a-411d-a329-d9554f488760\"}]},\"type\":\"ConnectorPlacement.EquallySpacedConnector\",\"uuid\":\"1e045dad-e983-4ca4-b515-afd5db4fa0f5\"}],\"packageUris\":[\"http://schema.mathworks.com/mf0/Connector/R2020b\"],\"version\":\"1.0\"}"
  Constant : Constant  Value=0
  MATLAB Function : MATLAB Function  TreatAsAtomicUnit=on
  Switch{,1..3} (4 alike) : Switch  Criteria=u2 > Threshold  SaturateOnIntegerOverflow=off  InputSameDT=off
  TorqueCm : Outport
  BrakeCm : Outport  Port=2
  tag scope: ActualAccel=global
  wires:
  Acceleration to Torque/2(brake_cm) -> BrakeCm/1, Switch2/3
  Acceleration to Torque/1(torque_cm) -> TorqueCm/1, Switch3/3
  ACCaccel_cmd/1 -> MATLAB Function/1(u)
  ACC/1 -> Switch1/2, Switch/2
  MATLAB Function/1(accel) -> Switch/1
  LCaccel_cmd/1 -> Acceleration to Torque/1(acc_cmd), Switch/3
  LCdeccel_cmd/1 -> Acceleration to Torque/2(decc_cmd), Switch1/3
  MATLAB Function/2(decel) -> Switch1/1
  Constant/1 -> Switch3/1
  Braking/1 -> Switch3/2, Switch2/2, Braking Command/4("Braking ")
  CurrVelocity/1 -> Braking Command/1(CurrVelocity)
  Relative Distance/1 -> Braking Command/2(Relative Distance)
  Braking Command/1(BrakeCm) -> Switch2/1
  CurrAccel/1 -> Braking Command/3(CurrAccel)
  Set Velocity/1 -> Braking Command/5(Set Velocity)
  HoldBrake/1 -> Braking Command/6(HoldBrake)
  Acceleration to Torque/3(ActualAccel) -> [ActualAccel]

== system ADC_RoadRunner/Environment & Data/BusActorPose To BusVehiclePose ==
  BusActorPose : Inport
  Bus Creator : BusCreator  Inputs=7  OutDataTypeStr=Bus: BusVehiclePose  NonVirtualBus=on
      settings: InheritFromInputs=off
  Bus Selector : BusSelector  OutputSignals=ActorID,Position,Velocity,Roll,Pitch,Yaw,AngularVelocity
  BusVehiclePose : Outport
  wires:
  BusActorPose/1 -> Bus Selector/1
  Bus Selector/1 -> Bus Creator/1  "<ActorID>"
  Bus Selector/2 -> Bus Creator/2  "<Position>"
  Bus Selector/4 -> Bus Creator/4  "<Roll>"
  Bus Selector/5 -> Bus Creator/5  "<Pitch>"
  Bus Selector/6 -> Bus Creator/6  "<Yaw>"
  Bus Selector/7 -> Bus Creator/7  "<AngularVelocity>"
  Bus Selector/3 -> Bus Creator/3  "<Velocity>"
  Bus Creator/1 -> BusVehiclePose/1

== system ADC_RoadRunner/Environment & Data/Calculate Norm ==
  Lateral Velocity : Inport
  Longitudinal Velocity : Inport  Port=2
  Add : Sum
  Math Function : Math  Operator=square
  Math Function1 : Math  Operator=square
  Sqrt : Sqrt
  Speed : Outport
  wires:
  Add/1 -> Sqrt/1
  Math Function1/1 -> Add/2
  Math Function/1 -> Add/1
  Sqrt/1 -> Speed/1
  Lateral Velocity/1 -> Math Function/1
  Longitudinal Velocity/1 -> Math Function1/1

== system ADC_RoadRunner/Environment & Data/ENU to NWD ==
  RR Position : Inport
  2D RefWaypoints : MATLAB Function  TreatAsAtomicUnit=on
  Gain : Gain  Gain=-1
  Matrix Concatenate : Concatenate  NumInputs=3  Mode=Multidimensional array  ConcatenateDimension=2
  Selector : Selector  NumberOfDimensions=2  InputPortWidth=3  IndexOptions=Select all,Index vector (dialog)  Indices=[1 3],1  OutputSizes=1,1
  Selector1 : Selector  NumberOfDimensions=2  InputPortWidth=3  IndexOptions=Select all,Index vector (dialog)  Indices=[1 3],2  OutputSizes=1,1
  Selector2 : Selector  NumberOfDimensions=2  InputPortWidth=3  IndexOptions=Select all,Index vector (dialog)  Indices=[1 3],3  OutputSizes=1,1
  Trajectory Waypoints : ToWorkspace  VariableName=Trajectory_Waypoints  SaveFormat=Structure  SampleTime=-1
      settings: Save2DSignal=2-D array (concatenate along first dimension)
  Cuboid Position : Outport
  Destination : Outport  Port=2
  Waypoints : Outport  Port=3
  Initial Position : Outport  Port=4
  Initial Yaw : Outport  Port=5
  wires:
  Gain/1 -> Matrix Concatenate/2
  Selector1/1 -> Matrix Concatenate/1
  Selector2/1 -> Matrix Concatenate/3
  Selector/1 -> Gain/1
  RR Position/1 -> Selector/1, Selector1/1, Selector2/1
  Matrix Concatenate/1 -> Cuboid Position/1, 2D RefWaypoints/1(trajectory)
  2D RefWaypoints/4(Destination_Position) -> Destination/1
  2D RefWaypoints/1(Trajectory_Waypoints) -> Trajectory Waypoints/1, Waypoints/1
  2D RefWaypoints/3(Initial_Position) -> Initial Position/1
  2D RefWaypoints/2(Initial_Yaw) -> Initial Yaw/1
